simulink model "extremumSeekingMfc"  (R2015a)
settings: Solver=ode15s  StartTime=0.0  StopTime=120  RelTol=1e-9  AbsTol=1e-12
InitFcn:
  | mfcInit = [20.8395 498.2432 2.0000 0.0412];
  | 
  | s0 = 300;
  | 
  | ap = 10;
  | unitEvalTime = 0.8;
  | unitFreq = 1 / unitEvalTime;
  | %wp = unitFreq / 10;
  | wp = 0.001;
  | wl = wp / 5;
  | wh = wl;
  | k  = 5;
  | Rinit = 20;
  | 
  | 
  | 
  | s0 = 600;
  | ap = 5;
  | wp = 1/5*2*pi;
  | wl = 0.26;
  | wh = .26;
  | k = 1200;
settings Model: Creator=ironi  LastModifiedBy=ironi
settings HardwareCC: ProdBitPerLong=64  ProdBitPerPointer=64  ProdWordSize=64  ProdHWDeviceType=Generic->64-bit Embedded Processor (LP64)

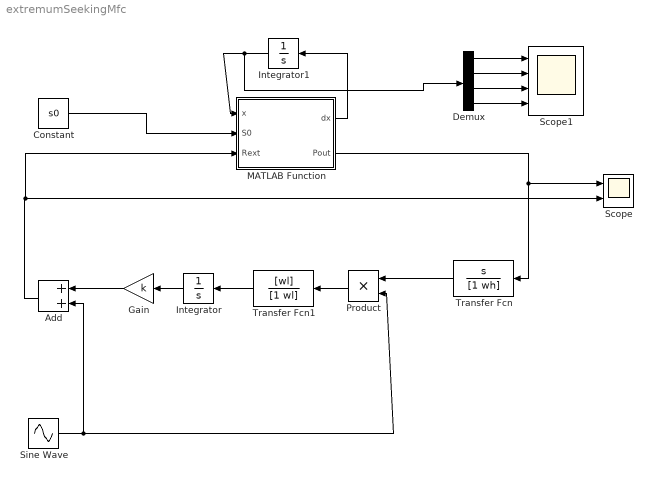
== system extremumSeekingMfc ==
  Add : Sum
  Constant : Constant  Value=s0
  Demux : Demux
  Gain : Gain  Gain=k
  Integrator : Integrator  InitialCondition=50/k
  Integrator1 : Integrator  InitialCondition=mfcInit
  MATLAB Function : MATLAB Function  TreatAsAtomicUnit=on
  Product : Product
  Scope : Scope  NumInputPorts=2
      settings: YMin=-5~-5  YMax=5~5
  Scope1 : Scope  NumInputPorts=4
      settings: YMin=-5~-5~-5~-5  YMax=5~5~5~5
  Sine Wave : Sin  Amplitude=ap  Frequency=wp  SampleTime=0
  Transfer Fcn : TransferFcn  Numerator=[1 0]  Denominator=[1 wh]
  Transfer Fcn1 : TransferFcn  Numerator=[wl]  Denominator=[1 wl]
  wires:
  Gain/1 -> Add/1
  Integrator/1 -> Gain/1
  Transfer Fcn1/1 -> Integrator/1
  Product/1 -> Transfer Fcn1/1
  Transfer Fcn/1 -> Product/1
  Sine Wave/1 -> Add/2, Product/2
  Add/1 -> MATLAB Function/3(Rext), Scope/2
  MATLAB Function/2(Pout) -> Scope/1, Transfer Fcn/1
  Constant/1 -> MATLAB Function/2(S0)
  MATLAB Function/1(dx) -> Integrator1/1
  Integrator1/1 -> Demux/1, MATLAB Function/1(x)
  Demux/4 -> Scope1/4
  Demux/3 -> Scope1/3
  Demux/1 -> Scope1/1
  Demux/2 -> Scope1/2

== matlab function extremumSeekingMfc/MATLAB Function ==
  data: dx output; x input; S0 input; Rext input; Pout output
function [dx, Pout] = mfcModel(x, S0, Rext)
F = 96485;
R = 8.314472;
T = 298.15;
Y = 22.753;
Ych4 = .3;
qmax_a = 8.48;
qmax_m = 8.2;
umax_a = 1.9753;
umax_m = .1;
Ks_a = 20;
Ks_m = 80;
m = 2;
gamma = 663400;
Mtotal = .05;
Km = .2*Mtotal;
Kd_a = .02*umax_a;
Kd_m = .02*umax_m;
Xmax_a = 512.5;
Xmax_m = 537.5;
Kx = .04;
Rmin = 25;
Rmax = 2000 + Rmin;
Emin = .01;
Emax = 0.25 + 0.4144+ Emin;
Kr = .024;

i0ref=0.4*4;

e = 0.0001*Mtotal;

V = 0.05;
Fin = 0.1527;

D = Fin/V;

S   = x(1);
xa  = x(2);
xm  = x(3);
Mox = x(4);

%% Équations dynamiques
  
Mred = Mtotal - Mox;

Rint = Rmin + (Rmax - Rmin) * exp(-Kr*xa);                          % (22)
Eocv = Emin + (Emax - Emin) * exp(-1/(Kr*xa));                      % (23)

alpha_a = 1/2*(1 + tanh(Kx*(xa + xm - Xmax_a)));                    % (9)
alpha_m = 1/2*(1 + tanh(Kx*(xa + xm - Xmax_m)));                    % (9)

qa = qmax_a * S / (Ks_a + S) * Mox / (Km + Mox);                    % (15)
qm = qmax_m * S / (Ks_m + S);                                       % (16)

ua = umax_a * S / (Ks_a + S) * Mox / (Km + Mox);                    % (13)
um = umax_m * S / (Ks_m + S);                                       % (14)

n_conc = R*T/F/m * log(Mtotal/Mred);                                % (18)

Imfc = (Eocv - n_conc) / (Rext + Rint) * Mred / (e + Mred);         % (21)

Sp = -qa*xa - qm*xm + D*(S0 - S);                                   % (6)
Xap = ua*xa - Kd_a*xa - alpha_a*D*xa;                               % (7)
Xmp = um*xm - Kd_m*xm - alpha_m*D*xm;                               % (8)

Moxp = -Y*qa + gamma*Imfc / (m*F*V*xa) * 86400;                     % (12)

if xa < 1 && Xap < 0
  Xap = 0;
end

if xm < 0.99 && Xmp < 0
  Xmp = 0;
end

Pout = Rext*Imfc^2;

dx = [Sp; Xap; Xmp; Moxp];
